simulink model "lab5_ASP_VoronkovM"  (R2018b)
settings: Solver=VariableStepAuto  StartTime=0.0  StopTime=10.0  RelTol=1e-3
libraries: dspsnks4 x1, dspvision x1
settings Model: Creator=Student  LastModifiedBy=Student

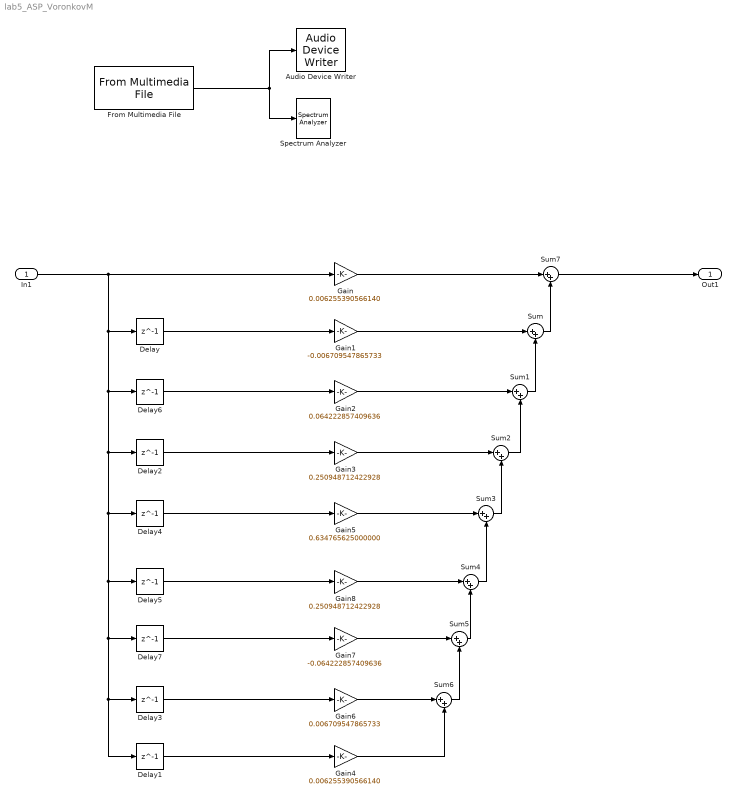
== system lab5_ASP_VoronkovM ==
  In1 : Inport
  Audio Device Writer : dspsnks4/Audio Device Writer  Driver=DirectSound  Device=Default  InheritSampleRate=on  SampleRate=44100  BitDepth=16-bit integer  BufferSize=4096  NumBuffers=10  DefaultOutputChannelMapping=on  OutputChannelMapping=1:2  OutputNumUnderrunSamples=off  DriverIdx=1  DeviceWarnFlag=''
  Delay{,1..7} (8 alike) : Delay  DelayLength=1  InitialCondition=0
  From Multimedia File : dspvision/From Multimedia File  inputFilename=C:\Users\student\Documents\MATLAB\song.mp3  loop=on  numPlays=inf  outputStreams=Audio only  videoDataType=single  audioDataType=double  inheritSampleTime=on  userDefinedSampleTime=1/30  noAudioOutput=off  isIntensityVideo=off  fourcc=RGB  colorVideoFormat=Separate color signals  outputEOF=off  dataOrg=Column-major  audioFrameSize=1024  computeAudioFrameSize=off  outSamplingMode=Sample based
      settings: SourceProductBaseCode=VP
  Gain : Gain  Gain=0.006255390566140
  Gain1 : Gain  Gain=-0.006709547865733
  Gain2 : Gain  Gain=0.064222857409636
  Gain3 : Gain  Gain=0.250948712422928
  Gain4 : Gain  Gain=0.006255390566140
  Gain5 : Gain  Gain=0.634765625000000
  Gain6 : Gain  Gain=0.006709547865733
  Gain7 : Gain  Gain=-0.064222857409636
  Gain8 : Gain  Gain=0.250948712422928
  Spectrum Analyzer : SpectrumAnalyzer
  Sum{,1..7} (8 alike) : Sum  Inputs=|++
  Out1 : Outport
  wires:
  From Multimedia File/1 -> Audio Device Writer/1, Spectrum Analyzer/1
  In1/1 -> Gain/1, Delay/1, Delay5/1, Delay7/1, Delay3/1, Delay1/1, Delay4/1, Delay2/1, Delay6/1
  Delay/1 -> Gain1/1
  Delay5/1 -> Gain8/1
  Delay4/1 -> Gain5/1
  Delay2/1 -> Gain3/1
  Delay6/1 -> Gain2/1
  Delay7/1 -> Gain7/1
  Delay3/1 -> Gain6/1
  Delay1/1 -> Gain4/1
  Gain1/1 -> Sum/1
  Gain2/1 -> Sum1/1
  Gain3/1 -> Sum2/1
  Gain5/1 -> Sum3/1
  Gain8/1 -> Sum4/1
  Gain7/1 -> Sum5/1
  Gain6/1 -> Sum6/1
  Gain4/1 -> Sum6/2
  Sum6/1 -> Sum5/2
  Sum5/1 -> Sum4/2
  Sum4/1 -> Sum3/2
  Sum3/1 -> Sum2/2
  Sum2/1 -> Sum1/2
  Sum1/1 -> Sum/2
  Sum/1 -> Sum7/2
  Gain/1 -> Sum7/1
  Sum7/1 -> Out1/1
